simulink model "fv_sim"  (R2021b)
settings: Solver=VariableStepAuto  StartTime=0.0  StopTime=10  RelTol=1e-3
values from neighbouring files (symbols this model uses):
  euler_angles_NfromB_0_deg = [0; 0; 0]    [run_simulation.m]
  euler_angles_NfromB_0_rad = deg2rad(euler_angles_NfromB_0_deg)    [run_simulation.m]
  EvB_BfromE_mps = [0; 0; 0]    [run_simulation.m]
  ExE_BfromE_0_m = lla2ecef([lat_d, lon_d, ground_level_m + altitude_m])'    [run_simulation.m]
  g_mps2 = 9.81    [run_simulation.m]
  J_kgm2 = [J_xx, J_xy, J_xz ... (first row only)    [get_mass_props.m]
  ll_NfromE_deg = [lat_d, lon_d]    [run_simulation.m]
  m_kg = sum(cmg(:,1))    [get_mass_props.m]
  omega_BwrtI_rps_0 = omega_BwrtN_rps + omega_EwrtI_rps_0    [run_simulation.m]
  omega_BwrtN_rps = deg2rad(omega_BwrtN_dps)    [run_simulation.m]
  re_m = 6378000    [run_simulation.m]
undefined symbols (not defined in the file or in its folder): quat_rate_IC
libraries: coordinate_transforms x16, aerolibutil x5, aerolibconvert2 x5, aerolibfltsims x4, simulink_extras x2, sharedutil x1, aerolibanimutils x1, aerodynamics x1, kinematics x1, vrlib x1
settings Model: Creator=Nikita  LastModifiedBy=Nikita
settings SolverCC: AlgebraicLoopSolver=TrustRegion
settings DebuggingCC: SFMachineParentedDataDiag=warning

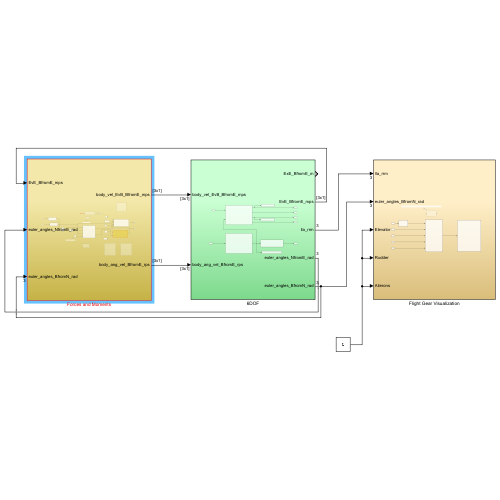
[thumbnail: Simulink's stored preview of the top-level diagram]
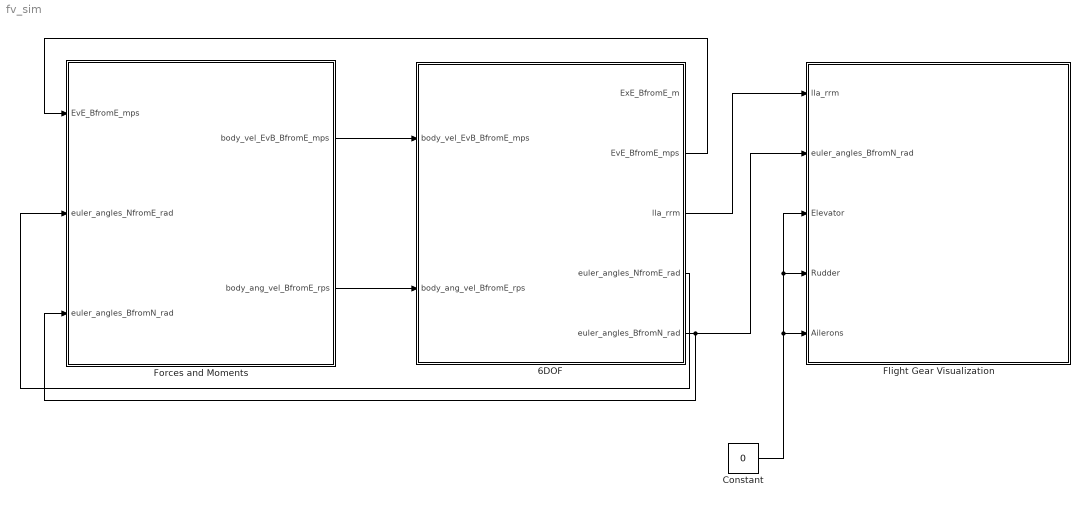
== system fv_sim ==
  6DOF : Subsystem
  Constant : Constant  Value=0
  Flight Gear Visualization : Subsystem
  Forces and Moments : Subsystem
  wires:
  6DOF/5(euler_angles_BfromN_rad) -> Forces and Moments/3(euler_angles_BfromN_rad), Flight Gear Visualization/2(euler_angles_BfromN_rad)
  Forces and Moments/1(body_vel_EvB_BfromE_mps) -> 6DOF/1(body_vel_EvB_BfromE_mps)
  Forces and Moments/2(body_ang_vel_BfromE_rps) -> 6DOF/2(body_ang_vel_BfromE_rps)
  6DOF/3(lla_rrm) -> Flight Gear Visualization/1(lla_rrm)
  Constant/1 -> Flight Gear Visualization/5(Ailerons), Flight Gear Visualization/4(Rudder), Flight Gear Visualization/3(Elevator)
  6DOF/4(euler_angles_NfromE_rad) -> Forces and Moments/2(euler_angles_NfromE_rad)
  6DOF/2(EvE_BfromE_mps) -> Forces and Moments/1(EvE_BfromE_mps)

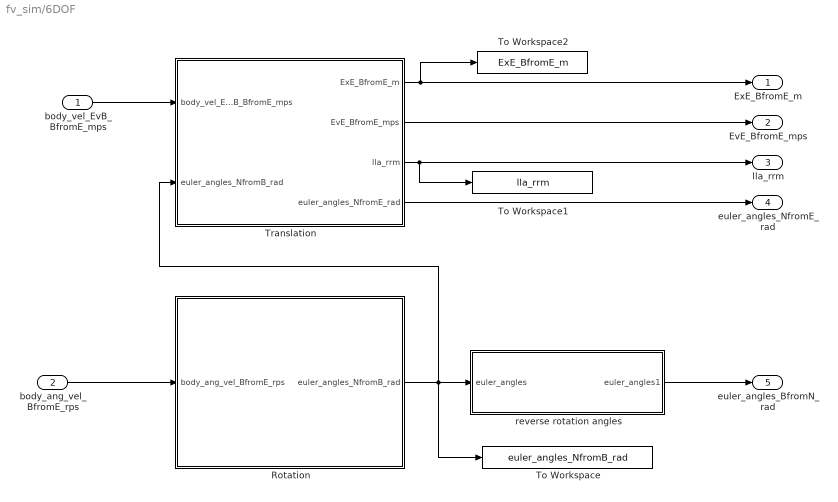
== system fv_sim/6DOF ==
  body_vel_EvB_BfromE_mps : Inport
  body_ang_vel_BfromE_rps : Inport  Port=2
  Rotation : Subsystem
  To Workspace : ToWorkspace  VariableName=euler_angles_NfromB_rad  SampleTime=-1
  To Workspace1 : ToWorkspace  VariableName=lla_rrm  SampleTime=-1
  To Workspace2 : ToWorkspace  VariableName=ExE_BfromE_m  SampleTime=-1
  Translation : Subsystem
  reverse rotation angles : Subsystem
  ExE_BfromE_m : Outport
  EvE_BfromE_mps : Outport  Port=2
  lla_rrm : Outport  Port=3
  euler_angles_NfromE_rad : Outport  Port=4
  euler_angles_BfromN_rad : Outport  Port=5
  wires:
  Translation/3(lla_rrm) -> lla_rrm/1, To Workspace1/1
  Translation/1(ExE_BfromE_m) -> ExE_BfromE_m/1, To Workspace2/1
  Translation/2(EvE_BfromE_mps) -> EvE_BfromE_mps/1
  reverse rotation angles/1(euler_angles1) -> euler_angles_BfromN_rad/1
  Rotation/1(euler_angles_NfromB_rad) -> reverse rotation angles/1(euler_angles), To Workspace/1, Translation/2(euler_angles_NfromB_rad)
  Translation/4(euler_angles_NfromE_rad) -> euler_angles_NfromE_rad/1
  body_vel_EvB_BfromE_mps/1 -> Translation/1(body_vel_EvB_BfromE_mps)
  body_ang_vel_BfromE_rps/1 -> Rotation/1(body_ang_vel_BfromE_rps)

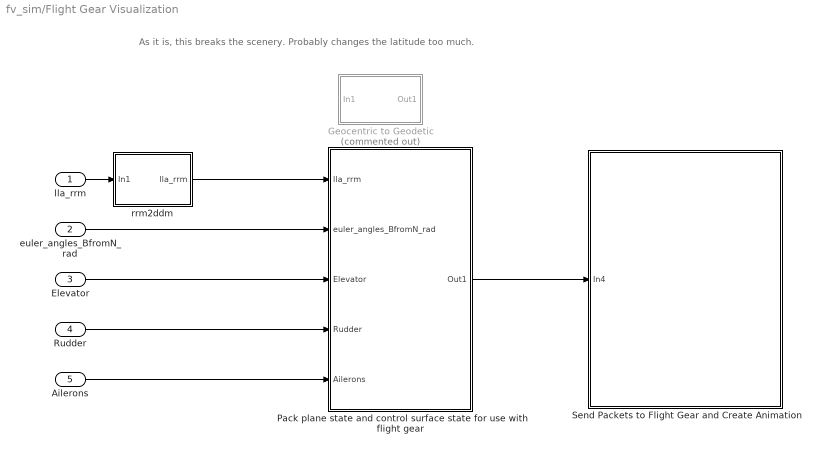
== system fv_sim/Flight Gear Visualization ==
  note: As it is, this breaks the scenery. Probably changes the latitude too much.
  lla_rrm : Inport
  euler_angles_BfromN_rad : Inport  Port=2
  Elevator : Inport  Port=3
  Rudder : Inport  Port=4
  Ailerons : Inport  Port=5
  Geocentric to Geodetic : Subsystem  Commented=on
  Pack plane state and control surface state for use with flight gear : Subsystem
  Send Packets to Flight Gear and Create Animation : Subsystem
  rrm2ddm : Subsystem
  wires:
  lla_rrm/1 -> rrm2ddm/1(In1)
  rrm2ddm/1(lla_rrm) -> Pack plane state and control surface state for use with flight gear/1(lla_rrm)
  euler_angles_BfromN_rad/1 -> Pack plane state and control surface state for use with flight gear/2(euler_angles_BfromN_rad)
  Elevator/1 -> Pack plane state and control surface state for use with flight gear/3(Elevator)
  Rudder/1 -> Pack plane state and control surface state for use with flight gear/4(Rudder)
  Ailerons/1 -> Pack plane state and control surface state for use with flight gear/5(Ailerons)
  Pack plane state and control surface state for use with flight gear/1(Out1) -> Send Packets to Flight Gear and Create Animation/1(In4)

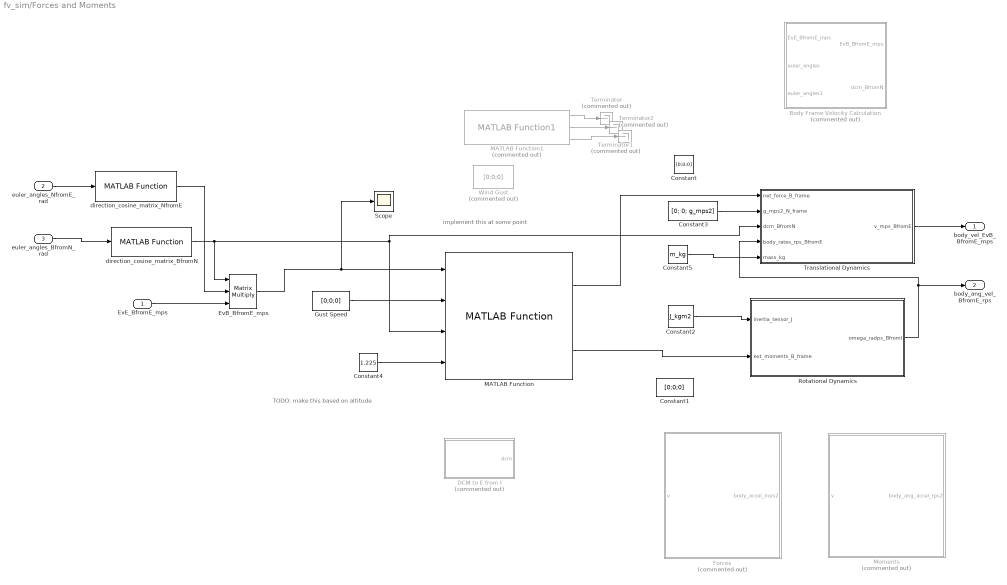
== system fv_sim/Forces and Moments ==
  note: TODO: make this based on altitude
  note: implement this at some point
  EvE_BfromE_mps : Inport
  euler_angles_NfromE_rad : Inport  Port=2
  euler_angles_BfromN_rad : Inport  Port=3
  Body Frame Velocity Calculation : Subsystem  Commented=on
  Constant : Constant  Value=[0;0;0]
  Constant1 : Constant  Value=[0;0;0]
  Constant2 : Constant  Value=J_kgm2
  Constant3 : Constant  Value=[0; 0; g_mps2]
  Constant4 : Constant  Value=1.225
  Constant5 : Constant  Value=m_kg
  DCM to E from I : Subsystem  Commented=on
  EvB_BfromE_mps : Product  Inputs=3  Multiplication=Matrix(*)
  Forces : Subsystem  Commented=on
  Gust Speed : Constant  Value=[0;0;0]
  MATLAB Function : aerodynamics/MATLAB Function  SystemSampleTime=-1  VariantActivationTime=update diagram  Latency=0  AutoFrameSizeCalculation=off
  MATLAB Function1 : kinematics/MATLAB Function1  Commented=on  SystemSampleTime=-1  VariantActivationTime=update diagram  Latency=0  AutoFrameSizeCalculation=off
  Moments : Subsystem  Commented=on
  Rotational Dynamics : Subsystem
  Scope : Scope
  Terminator : Terminator  Commented=on
  Terminator1 : Terminator  Commented=on
  Terminator2 : Terminator  Commented=on
  Translational Dynamics : Subsystem
  Wind Gust : Constant  Commented=on  Value=[0;0;0]
  direction_cosine_matrix_BfromN : coordinate_transforms/MATLAB Function  SystemSampleTime=-1  VariantActivationTime=update diagram  Latency=0  AutoFrameSizeCalculation=off
  direction_cosine_matrix_NfromE : coordinate_transforms/MATLAB Function  SystemSampleTime=-1  VariantActivationTime=update diagram  Latency=0  AutoFrameSizeCalculation=off
  body_vel_EvB_BfromE_mps : Outport
  body_ang_vel_BfromE_rps : Outport  Port=2
  wires:
  euler_angles_BfromN_rad/1 -> direction_cosine_matrix_BfromN/1
  Translational Dynamics/1(v_mps_BfromE) -> body_vel_EvB_BfromE_mps/1
  Rotational Dynamics/1(omega_radps_BfromI) -> body_ang_vel_BfromE_rps/1, Translational Dynamics/4(body_rates_rps_BfromE)
  Constant2/1 -> Rotational Dynamics/1(inertia_tensor_J)
  Constant3/1 -> Translational Dynamics/2(g_mps2_N_frame)
  direction_cosine_matrix_BfromN/1 -> EvB_BfromE_mps/1, MATLAB Function/3, Translational Dynamics/3(dcm_BfromN)
  ? -> MATLAB Function1/1
  Constant4/1 -> MATLAB Function/4
  Gust Speed/1 -> MATLAB Function/2
  MATLAB Function1/1 -> Terminator/1
  MATLAB Function1/2 -> Terminator1/1
  MATLAB Function1/3 -> Terminator2/1
  Constant5/1 -> Translational Dynamics/5(mass_kg)
  euler_angles_NfromE_rad/1 -> direction_cosine_matrix_NfromE/1
  direction_cosine_matrix_NfromE/1 -> EvB_BfromE_mps/2
  EvE_BfromE_mps/1 -> EvB_BfromE_mps/3
  EvB_BfromE_mps/1 -> MATLAB Function/1, Scope/1
  MATLAB Function/1 -> Translational Dynamics/1(net_force_B_frame)
  MATLAB Function/2 -> Rotational Dynamics/2(ext_moments_B_frame)

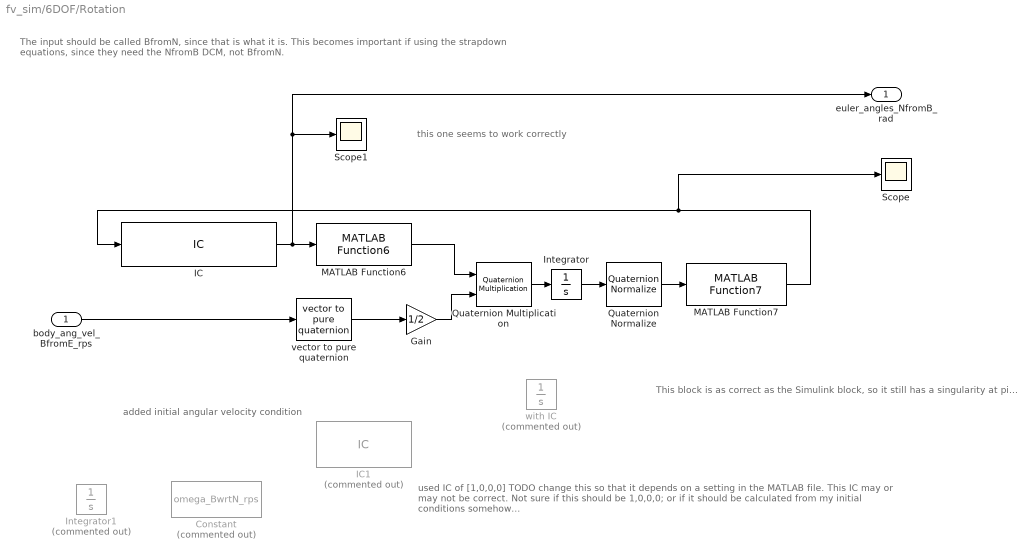
== system fv_sim/6DOF/Rotation ==
  note: this one seems to work correctly
  note: This block is as correct as the Simulink block, so it still has a singularity at pi...
  note: The input should be called BfromN, since that is what it is.
      |
      | This becomes important if using the strapdown equations, since they need the NfromB DCM, not BfromN.
  note: used IC of [1,0,0,0]
      | TODO change this so that it depends on a setting in the MATLAB file. This IC may or may not be correct.
      | Not sure if this should be 1,0,0,0; or if it should be calculated from my initial conditions somehow...
  note: added initial angular velocity condition
  body_ang_vel_BfromE_rps : Inport
  Constant : Constant  Commented=on  Value=omega_BwrtN_rps
  Gain : Gain  Gain=1/2
  IC : InitialCondition  Value=euler_angles_NfromB_0_rad
  IC1 : InitialCondition  Commented=on  Value=omega_BwrtN_rps
  Integrator : Integrator  InitialCondition=[1;0;0;0]
  Integrator1 : Integrator  Commented=on  InitialCondition=omega_BwrtN_rps
  MATLAB Function6 : coordinate_transforms/MATLAB Function6  SystemSampleTime=-1  VariantActivationTime=update diagram  Latency=0  AutoFrameSizeCalculation=off
  MATLAB Function7 : coordinate_transforms/MATLAB Function7  SystemSampleTime=-1  VariantActivationTime=update diagram  Latency=0  AutoFrameSizeCalculation=off
  Quaternion Multiplication : aerolibutil/Quaternion Multiplication
  Quaternion Normalize : sharedutil/Quaternion Normalize  aMode=aMode
      settings: SourceProductBaseCode=AE,PW,DR,MT,UV,VE
  Scope : Scope
  Scope1 : Scope
  vector to pure quaternion : coordinate_transforms/vector to pure quaternion  SystemSampleTime=-1  VariantActivationTime=update diagram  Latency=0  AutoFrameSizeCalculation=off
  with IC : Integrator  Commented=on  InitialCondition=quat_rate_IC
  euler_angles_NfromB_rad : Outport
  wires:
  Quaternion Multiplication/1 -> Integrator/1
  Gain/1 -> Quaternion Multiplication/2
  vector to pure quaternion/1 -> Gain/1
  Integrator/1 -> Quaternion Normalize/1
  IC/1 -> MATLAB Function6/1, Scope1/1, euler_angles_NfromB_rad/1
  MATLAB Function6/1 -> Quaternion Multiplication/1
  Quaternion Normalize/1 -> MATLAB Function7/1
  body_ang_vel_BfromE_rps/1 -> vector to pure quaternion/1
  MATLAB Function7/1 -> Scope/1, IC/1

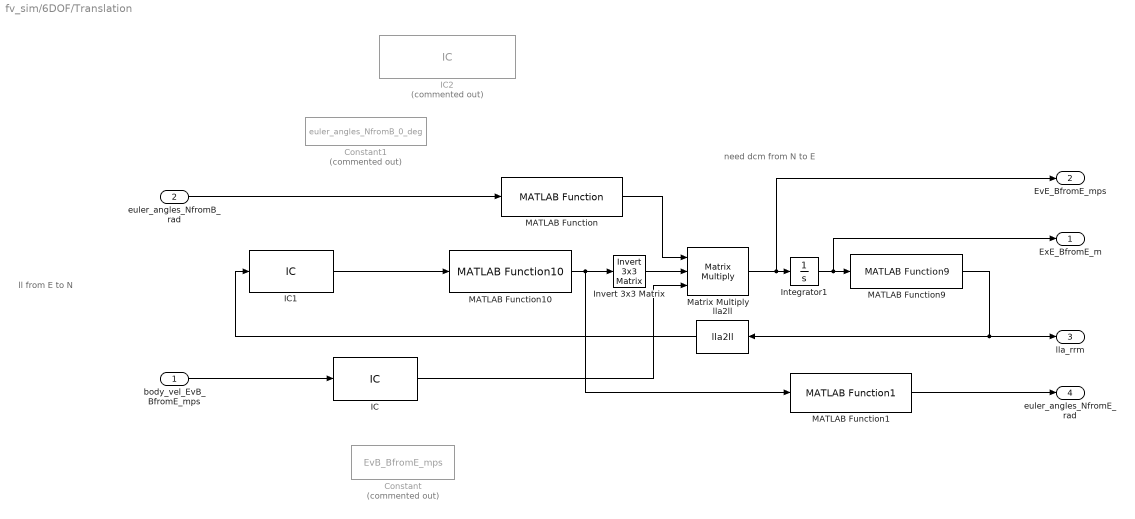
== system fv_sim/6DOF/Translation ==
  note: need dcm from N to E
  note: ll from E to N
  body_vel_EvB_BfromE_mps : Inport
  euler_angles_NfromB_rad : Inport  Port=2
  Constant : Constant  Commented=on  Value=EvB_BfromE_mps
  Constant1 : Constant  Commented=on  Value=euler_angles_NfromB_0_deg
  IC : InitialCondition  Value=EvB_BfromE_mps
  IC1 : InitialCondition  Value=ll_NfromE_deg
  IC2 : InitialCondition  Commented=on  Value=euler_angles_NfromB_0_deg
  Integrator1 : Integrator  InitialCondition=ExE_BfromE_0_m
  Invert 3x3 Matrix : aerolibutil/Invert  3x3 Matrix
  MATLAB Function : coordinate_transforms/MATLAB Function  SystemSampleTime=-1  VariantActivationTime=update diagram  Latency=0  AutoFrameSizeCalculation=off
  MATLAB Function1 : coordinate_transforms/MATLAB Function1  SystemSampleTime=-1  VariantActivationTime=update diagram  Latency=0  AutoFrameSizeCalculation=off
  MATLAB Function10 : coordinate_transforms/MATLAB Function10  SystemSampleTime=-1  VariantActivationTime=update diagram  Latency=0  AutoFrameSizeCalculation=off
  MATLAB Function9 : coordinate_transforms/MATLAB Function9  SystemSampleTime=-1  VariantActivationTime=update diagram  Latency=0  AutoFrameSizeCalculation=off
  Matrix Multiply : Product  Inputs=3  Multiplication=Matrix(*)
  lla2ll : coordinate_transforms/lla2ll  SystemSampleTime=-1  VariantActivationTime=update diagram  Latency=0  AutoFrameSizeCalculation=off
  ExE_BfromE_m : Outport
  EvE_BfromE_mps : Outport  Port=2
  lla_rrm : Outport  Port=3
  euler_angles_NfromE_rad : Outport  Port=4
  wires:
  MATLAB Function/1 -> Matrix Multiply/1
  Integrator1/1 -> ExE_BfromE_m/1, MATLAB Function9/1
  lla2ll/1 -> IC1/1
  Invert 3x3 Matrix/1 -> Matrix Multiply/2
  MATLAB Function9/1 -> lla2ll/1, lla_rrm/1
  Matrix Multiply/1 -> EvE_BfromE_mps/1, Integrator1/1
  IC1/1 -> MATLAB Function10/1
  MATLAB Function10/1 -> MATLAB Function1/1, Invert 3x3 Matrix/1
  MATLAB Function1/1 -> euler_angles_NfromE_rad/1
  euler_angles_NfromB_rad/1 -> MATLAB Function/1
  body_vel_EvB_BfromE_mps/1 -> IC/1
  IC/1 -> Matrix Multiply/3

== system fv_sim/6DOF/reverse rotation angles ==
  note: converting to Euler angles from N to B since that is more useful outside of here
  euler_angles : Inport
  Invert 3x3 Matrix : aerolibutil/Invert  3x3 Matrix
  MATLAB Function : coordinate_transforms/MATLAB Function  SystemSampleTime=-1  VariantActivationTime=update diagram  Latency=0  AutoFrameSizeCalculation=off
  MATLAB Function1 : coordinate_transforms/MATLAB Function1  SystemSampleTime=-1  VariantActivationTime=update diagram  Latency=0  AutoFrameSizeCalculation=off
  euler_angles1 : Outport
  wires:
  MATLAB Function/1 -> Invert 3x3 Matrix/1
  Invert 3x3 Matrix/1 -> MATLAB Function1/1
  MATLAB Function1/1 -> euler_angles1/1
  euler_angles/1 -> MATLAB Function/1

== system fv_sim/Flight Gear Visualization/Geocentric to Geodetic ==
  In1 : Inport
  Constant1 : Constant  Value=re_m
  Demux : Demux  Outputs=3
  Geocentric to Geodetic Latitude : Geoc2Geod
  Mux2 : Mux  Inputs=3
  Sum : Sum  Inputs=|++
  Out1 : Outport
  wires:
  Constant1/1 -> Sum/2
  Geocentric to Geodetic Latitude/1 -> Mux2/1
  Demux/3 -> Mux2/3, Sum/1
  Demux/1 -> Geocentric to Geodetic Latitude/1
  Sum/1 -> Geocentric to Geodetic Latitude/2
  Demux/2 -> Mux2/2
  In1/1 -> Demux/1
  Mux2/1 -> Out1/1

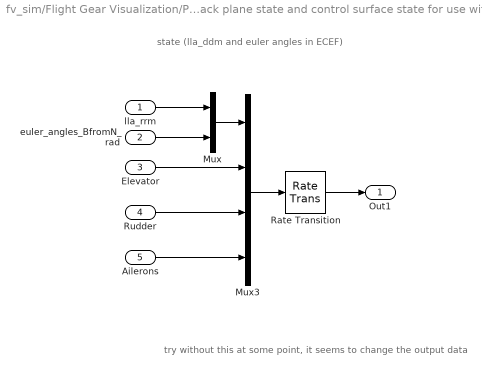
== system fv_sim/Flight Gear Visualization/Pack plane state and control surface state for use with flight gear ==
  note: try without this at some point, it seems to change the output data
  note: state (lla_ddm and euler angles in ECEF)
  lla_rrm : Inport
  euler_angles_BfromN_rad : Inport  Port=2
  Elevator : Inport  Port=3
  Rudder : Inport  Port=4
  Ailerons : Inport  Port=5
  Mux : Mux  Inputs=2
  Mux3 : Mux
  Rate Transition : RateTransition  Integrity=off  OutPortSampleTime=1/30
  Out1 : Outport
  wires:
  Ailerons/1 -> Mux3/4
  euler_angles_BfromN_rad/1 -> Mux/2
  Rudder/1 -> Mux3/3
  Mux/1 -> Mux3/1
  Mux3/1 -> Rate Transition/1
  Elevator/1 -> Mux3/2
  Rate Transition/1 -> Out1/1
  lla_rrm/1 -> Mux/1

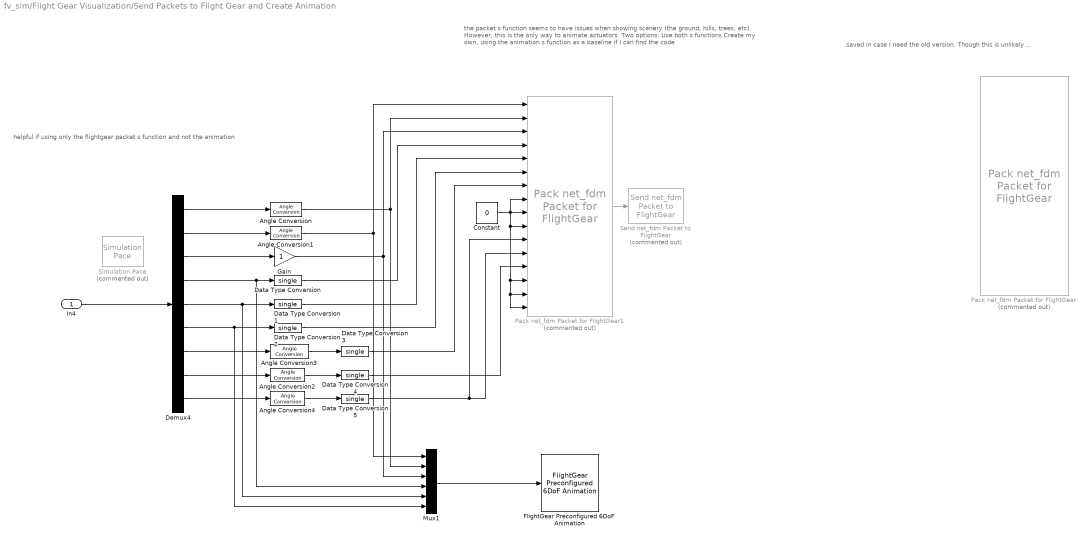
== system fv_sim/Flight Gear Visualization/Send Packets to Flight Gear and Create Animation ==
  note: the packet s function seems to have issues when showing scenery (the ground, hills, trees, etc). However, this is the only way to animate actuators. Two options:
      | Use both s functions
      | Create my own, using the animation s function as a baseline if I can find the code
  note: saved in case I need the old version. Though this is unlikely...
  note: helpful if using only the flightgear packet s function and not the animation
  In4 : Inport
  Angle Conversion : aerolibconvert2/Angle Conversion  IU=deg  OU=rad
  Angle Conversion1 : aerolibconvert2/Angle Conversion  IU=deg  OU=rad
  Angle Conversion2 : aerolibconvert2/Angle Conversion  IU=rad  OU=deg
  Angle Conversion3 : aerolibconvert2/Angle Conversion  IU=rad  OU=deg
  Angle Conversion4 : aerolibconvert2/Angle Conversion  IU=rad  OU=deg
  Constant : Constant  Value=0
  Data Type Conversion{,1..5} (6 alike) : DataTypeConversion  OutDataTypeStr=single
  Demux4 : Demux  Outputs=9
  FlightGear Preconfigured 6DoF Animation : aerolibfltsims/FlightGear Preconfigured 6DoF Animation  xFlightGearVersion=v2019.1  DestinationIpAddress=127.0.0.1  DestinationPort=5502  SampleTime=1/30  packetVersion=24
  Gain : Gain
  Mux1 : Mux  Inputs=6
  Pack net_fdm Packet for FlightGear : aerolibfltsims/Pack net_fdm Packet for FlightGear  Commented=on  FlightGearVersion=v2019.1  ShowPositionAttitudeInputs=on  ShowVelocityAccelerationInputs=off  ShowControlSurfacePositionInputs=on  ShowEngineFuelInputs=off  ShowLandingGearInputs=off  ShowEnvironmentInputs=off  SampleTime=1/30  packetVersion=24
      settings: SourceProductBaseCode=AE
  Pack net_fdm Packet for FlightGear1 : aerolibfltsims/Pack net_fdm Packet for FlightGear  Commented=on  FlightGearVersion=v2019.1  ShowPositionAttitudeInputs=on  ShowVelocityAccelerationInputs=off  ShowControlSurfacePositionInputs=on  ShowEngineFuelInputs=off  ShowLandingGearInputs=off  ShowEnvironmentInputs=off  SampleTime=1/30  packetVersion=24
      settings: SourceProductBaseCode=AE
  Send net_fdm Packet to FlightGear : aerolibfltsims/Send net_fdm Packet to FlightGear  Commented=on  DestinationIpAddress=127.0.0.1  DestinationPort=5502  LocalIpPort=-1  varLen=off  SampleTime=1/30
      settings: SourceProductBaseCode=AE
  Simulation Pace : aerolibanimutils/Simulation Pace  Commented=on  SimulationPace=1  SleepMode=MATLAB Thread  OutputPaceError=off  SampleTime=1/30
      settings: AttributesFormatString=%<SimulationPace> sec/sec
  wires:
  Data Type Conversion2/1 -> Pack net_fdm Packet for FlightGear1/6
  Mux1/1 -> FlightGear Preconfigured 6DoF Animation/1
  Angle Conversion1/1 -> Mux1/1, Pack net_fdm Packet for FlightGear1/1
  Angle Conversion2/1 -> Data Type Conversion4/1
  Demux4/9 -> Angle Conversion4/1
  Angle Conversion3/1 -> Data Type Conversion3/1
  Gain/1 -> Pack net_fdm Packet for FlightGear1/3, Mux1/3
  Demux4/4 -> Mux1/4, Data Type Conversion/1
  Data Type Conversion5/1 -> Pack net_fdm Packet for FlightGear1/12, Pack net_fdm Packet for FlightGear1/11
  Angle Conversion/1 -> Mux1/2, Pack net_fdm Packet for FlightGear1/2
  In4/1 -> Demux4/1
  Demux4/6 -> Mux1/6, Data Type Conversion2/1
  Angle Conversion4/1 -> Data Type Conversion5/1
  Constant/1 -> Pack net_fdm Packet for FlightGear1/9, Pack net_fdm Packet for FlightGear1/8, Pack net_fdm Packet for FlightGear1/16, Pack net_fdm Packet for FlightGear1/15, Pack net_fdm Packet for FlightGear1/14, Pack net_fdm Packet for FlightGear1/10
  Data Type Conversion1/1 -> Pack net_fdm Packet for FlightGear1/5
  Data Type Conversion3/1 -> Pack net_fdm Packet for FlightGear1/7
  Data Type Conversion/1 -> Pack net_fdm Packet for FlightGear1/4
  Demux4/5 -> Mux1/5, Data Type Conversion1/1
  Demux4/3 -> Gain/1
  Demux4/1 -> Angle Conversion/1
  Demux4/2 -> Angle Conversion1/1
  Demux4/8 -> Angle Conversion2/1
  Data Type Conversion4/1 -> Pack net_fdm Packet for FlightGear1/13
  Demux4/7 -> Angle Conversion3/1
  Pack net_fdm Packet for FlightGear1/1 -> Send net_fdm Packet to FlightGear/1

== system fv_sim/Flight Gear Visualization/rrm2ddm ==
  In1 : Inport
  Demux : Demux  Outputs=3
  Mux1 : Mux  Inputs=3
  Radians to Degrees : simulink_extras/Transformations/Radians to Degrees
  Radians to Degrees1 : simulink_extras/Transformations/Radians to Degrees
  lla_rrm : Outport
  wires:
  Demux/1 -> Radians to Degrees/1
  Radians to Degrees/1 -> Mux1/1
  Mux1/1 -> lla_rrm/1
  Demux/2 -> Radians to Degrees1/1
  Demux/3 -> Mux1/3
  Radians to Degrees1/1 -> Mux1/2
  In1/1 -> Demux/1

== system fv_sim/Forces and Moments/Body Frame Velocity Calculation ==
  note: converting EvE velocity to EvB for drag calculation
  EvE_BfromE_mps : Inport
  euler_angles : Inport  Port=2
  euler_angles1 : Inport  Port=3
  Matrix Multiply : Product  Inputs=3  Multiplication=Matrix(*)
  dcm_NfromE : coordinate_transforms/MATLAB Function  SystemSampleTime=-1  VariantActivationTime=update diagram  Latency=0  AutoFrameSizeCalculation=off
  direction_cosine_matrix_BfromN : coordinate_transforms/MATLAB Function  SystemSampleTime=-1  VariantActivationTime=update diagram  Latency=0  AutoFrameSizeCalculation=off
  EvB_BfromE_mps : Outport
  dcm_BfromN : Outport  Port=2
  wires:
  Matrix Multiply/1 -> EvB_BfromE_mps/1
  EvE_BfromE_mps/1 -> Matrix Multiply/3
  direction_cosine_matrix_BfromN/1 -> dcm_BfromN/1, Matrix Multiply/1
  dcm_NfromE/1 -> Matrix Multiply/2
  euler_angles/1 -> direction_cosine_matrix_BfromN/1
  euler_angles1/1 -> dcm_NfromE/1

== system fv_sim/Forces and Moments/DCM to E from I ==
  note: angles to E from I
  Clock : Clock
  MATLAB Function : coordinate_transforms/MATLAB Function  SystemSampleTime=-1  Latency=0  AutoFrameSizeCalculation=off
  Product : Product
  rotation of Earth : Constant  Value=omega_BwrtI_rps_0
  dcm : Outport
  wires:
  Clock/1 -> Product/1
  Product/1 -> MATLAB Function/1
  rotation of Earth/1 -> Product/2
  MATLAB Function/1 -> dcm/1

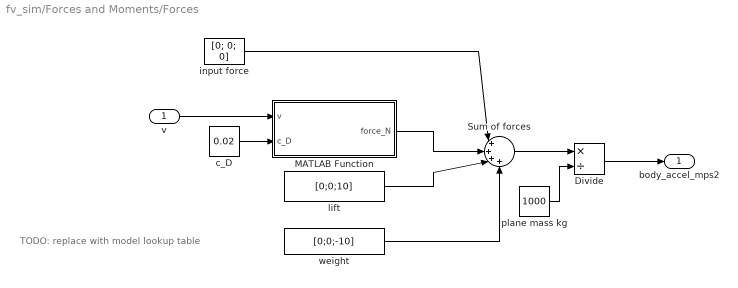
== system fv_sim/Forces and Moments/Forces ==
  note: TODO: replace with model lookup table
  v : Inport
  Divide : Product  Inputs=*/
  MATLAB Function : MATLAB Function  TreatAsAtomicUnit=on
  Sum of forces : Sum  Inputs=|++++
  c_D : Constant  Value=0.02
  input force : Constant  Value=[0; 0; 0]
  lift : Constant  Value=[0;0;10]
  plane mass kg : Constant  Value=1000
  weight : Constant  Value=[0;0;-10]
  body_accel_mps2 : Outport
  wires:
  input force/1 -> Sum of forces/1
  Divide/1 -> body_accel_mps2/1
  Sum of forces/1 -> Divide/1
  lift/1 -> Sum of forces/3
  MATLAB Function/1(force_N) -> Sum of forces/2
  c_D/1 -> MATLAB Function/2(c_D)
  v/1 -> MATLAB Function/1(v)
  weight/1 -> Sum of forces/4
  plane mass kg/1 -> Divide/2

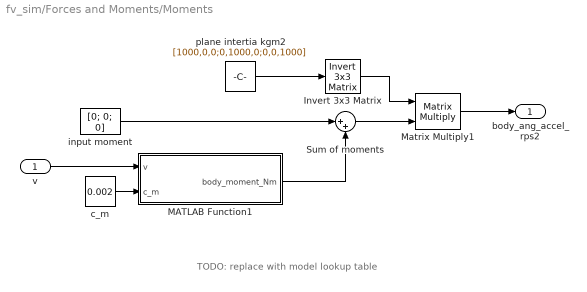
== system fv_sim/Forces and Moments/Moments ==
  note: TODO: replace with model lookup table
  v : Inport
  Invert 3x3 Matrix : aerolibutil/Invert  3x3 Matrix
  MATLAB Function1 : MATLAB Function  TreatAsAtomicUnit=on
  Matrix Multiply1 : Product  Multiplication=Matrix(*)
  Sum of moments : Sum  Inputs=|++
  c_m : Constant  Value=0.002
  input moment : Constant  Value=[0; 0; 0]
  plane intertia kgm2 : Constant  Value=[1000,0,0;0,1000,0;0,0,1000]
  body_ang_accel_rps2 : Outport
  wires:
  v/1 -> MATLAB Function1/1(v)
  Sum of moments/1 -> Matrix Multiply1/2
  Invert 3x3 Matrix/1 -> Matrix Multiply1/1
  Matrix Multiply1/1 -> body_ang_accel_rps2/1
  MATLAB Function1/1(body_moment_Nm) -> Sum of moments/2
  plane intertia kgm2/1 -> Invert 3x3 Matrix/1
  input moment/1 -> Sum of moments/1
  c_m/1 -> MATLAB Function1/2(c_m)

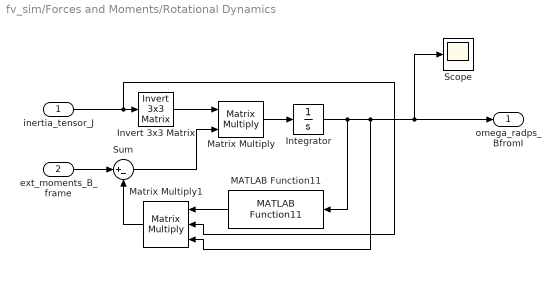
== system fv_sim/Forces and Moments/Rotational Dynamics ==
  inertia_tensor_J : Inport
  ext_moments_B_frame : Inport  Port=2
  Integrator : Integrator  InitialCondition=omega_BwrtI_rps_0
  Invert 3x3 Matrix : aerolibutil/Invert  3x3 Matrix
  MATLAB Function11 : coordinate_transforms/MATLAB Function11  SystemSampleTime=-1  VariantActivationTime=update diagram  Latency=0  AutoFrameSizeCalculation=off
  Matrix Multiply : Product  Multiplication=Matrix(*)
  Matrix Multiply1 : Product  Inputs=3  Multiplication=Matrix(*)
  Scope : Scope
  Sum : Sum  Inputs=|+-
  omega_radps_BfromI : Outport
  wires:
  Integrator/1 -> MATLAB Function11/1, Scope/1, omega_radps_BfromI/1, Matrix Multiply1/3
  inertia_tensor_J/1 -> Invert 3x3 Matrix/1, Matrix Multiply1/2
  Matrix Multiply1/1 -> Sum/2
  Invert 3x3 Matrix/1 -> Matrix Multiply/1
  MATLAB Function11/1 -> Matrix Multiply1/1
  Sum/1 -> Matrix Multiply/2
  ext_moments_B_frame/1 -> Sum/1
  Matrix Multiply/1 -> Integrator/1

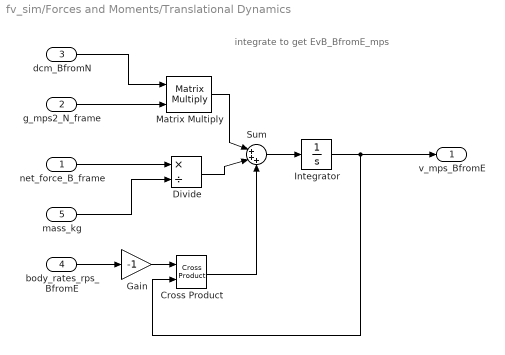
== system fv_sim/Forces and Moments/Translational Dynamics ==
  note: integrate to get EvB_BfromE_mps
  net_force_B_frame : Inport
  g_mps2_N_frame : Inport  Port=2
  dcm_BfromN : Inport  Port=3
  body_rates_rps_BfromE : Inport  Port=4
  mass_kg : Inport  Port=5
  Cross Product : vrlib/Utilities/Cross Product
  Divide : Product  Inputs=*/
  Gain : Gain  Gain=-1
  Integrator : Integrator  InitialCondition=EvB_BfromE_mps
  Matrix Multiply : Product  Multiplication=Matrix(*)
  Sum : Sum  Inputs=|+++
  v_mps_BfromE : Outport
  wires:
  g_mps2_N_frame/1 -> Matrix Multiply/2
  dcm_BfromN/1 -> Matrix Multiply/1
  Integrator/1 -> v_mps_BfromE/1, Cross Product/2
  Matrix Multiply/1 -> Sum/1
  net_force_B_frame/1 -> Divide/1
  Sum/1 -> Integrator/1
  Cross Product/1 -> Sum/3
  body_rates_rps_BfromE/1 -> Gain/1
  Gain/1 -> Cross Product/1
  mass_kg/1 -> Divide/2
  Divide/1 -> Sum/2

== matlab function fv_sim/Forces and Moments/Forces/MATLAB Function ==
  data: v input; force_N output; c_D input
% Input the velocity vector EvB_BfromE_mps and the total aircraft drag
% coefficient c_D
function force_N = aero_drag(v, c_D)

rho_kgpm3 = 1.225; % TODO replace with a constant
S = 20; % TODO replace with a value from a plane parameter file

% -0.5*r*v^2*S*c_D is scalar. Need to multiply by the v unit vector to get
% direction. norm(v)^2*v/norm(v) = norm(v)*v, therefore:
force_N = -1/2*rho_kgpm3*norm(v)*S*c_D*v;

== matlab function fv_sim/Forces and Moments/Moments/MATLAB Function1 ==
  data: v input; body_moment_Nm output; c_m input
% Input the velocity vector EvE_BfromE_mps and the total aircraft pitching
% moment coefficient, c_m
function body_moment_Nm = aero_drag_moment(v, c_m)

rho_kgpm3 = 1.225; % TODO replace with a constant
S = 20; % TODO replace with a value from a plane parameter file
c = 2; % chordlength

j_hat = [0; 1; 0]; % Unit vector in right (Y) direction in the body frame

% 0.5*r*v^2*S*c*c_m is scalar. Need to multiply by the unit vector in the
% right (Y) direction in the body frame.
body_moment_Nm = 1/2*rho_kgpm3*norm(v)^2*S*c*c_m*j_hat;
